simulink model "DvrSimKeybdCircuit_cs"  (R2016a)
settings: Solver=ode5  SolverMode=SingleTasking  StartTime=0.0  StopTime=inf  FixedStep=1/1000  RelTol=1e-3
PreLoadFcn:
  | mbxruntime.callbacks.PreLoadFcn(bdroot);
PostLoadFcn:
  | mbxruntime.callbacks.PostLoadFcn(bdroot);
InitFcn:
  | mbxruntime.callbacks.InitFcn(bdroot);
StartFcn:
  | mbxruntime.callbacks.StartFcn(bdroot);
StopFcn:
  | mbxruntime.callbacks.StopFcn(bdroot);
model workspace (MAT data in the model file):
  mbox_table : struct (value not decoded)
  model_closed = 0
  sim_status = 0
undefined symbols (not defined in the file or in its folder): BMotor1, BMotor2, BrkDelayTime, DControlB, Delay1, Delay2, DiscIntNeverNeededParam, IControlB, JMotor1, JMotor2, PControlB, PreScanCarSimLoadFcn, ratioGearF, ratioGearR, TorqDelayTime, Tstep
undefined symbols (not defined in the file): SteeringColumn, SteeringWheel, WheelL0, WheelL1, WheelR0, WheelR1
libraries: simulink x12, simulink_extras x5, MyLib x3, PreScanSimulinkLibrary x3, Solver_SF x2, pil_lib x1, PreScanUsefulBlocks x1
(part 4 of 9)

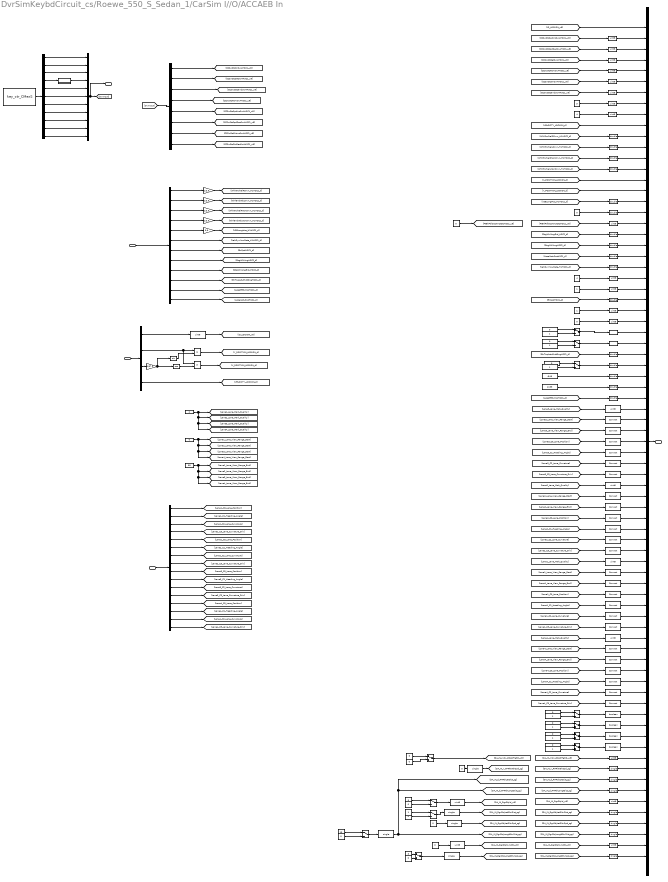
== system DvrSimKeybdCircuit_cs/Roewe_550_S_Sedan_1/CarSim I//O/ACCAEB In ==
  note: Here was constant 1, dont know why
  CarSimOut : Inport
  LanesInfo : Inport  Port=2
  LR_TIS : Inport  Port=3
  BrkPdlPos_H1HSC1_d1 : Constant  Value=0  OutDataTypeStr=double
  BrkPdlPos_H1HSC1_d2 : Constant  Value=0  OutDataTypeStr=uint8
  Bus Creator : BusCreator  Inputs=11
  Bus Creator1 : BusCreator  Inputs=77
  Bus Selector : BusSelector  OutputSignals=Lane1C0,Lane1C1,Lane1C2,Lane1C3,Lane2C0,Lane2C1,Lane2C2,Lane2C3,Lane3C0,Lane3C1,Lane3C2,Lane3C3,Lane4C0,Lane4C1,Lane4C2,Lane4C3
  Bus Selector1 : BusSelector  OutputSignals=WhlGndVelRDrvn_H1HSC2_d[km/h] (signal 38),WhlGndVelLDrvn_H1HSC2_d[km/h] (signal 39),WhlGndVelRNonDrvn_H1HSC2_d[km/h] (signal 40),WhlGndVelLNonDrvn_H1HSC2_d[km/h] (signal 41),VSELongtAcc_H1HSC1_d[g] (signal 42),VehDynYawRate_H1HSC1_d[deg/s] (signal 43),EnSpdHSC1_d[rpm] (signal 36),SteeringWheelAngle[deg] (signal 34),StrgWhlAngGrd_HSC2_d[deg/s] (signal 44),EnToqActuExtdRngHSC1_d[N M] (signal 37),AccelEfctvPosHSC1_d (signal 46),AccelActuPosHSC1_d (signal 45)
  Bus Selector2 : BusSelector  OutputSignals=ID ,Range ,Theta ,RlvSpd
  Bus Selector4 : BusSelector  OutputSignals=On,Set,Cancel,Resume,SpdInc,SpdDec,DisInc,DisDec
  Constant : Constant  Value=2
  Constant{1,93,102,104..105,107,110..111} (8 alike) : Constant  Value=0
  Constant{94,103,106,108..109,112..113} (7 alike) : Constant
  Constant2 : Constant  Value=95
  Constant3 : Constant  Value=1199
  Constant4 : Constant  Value=-848
  DA_IN_DgrObjSyncCtr_u1 : Constant  Value=0  OutDataTypeStr=uint8
  DA_IN_DgrObjSyncCtr_u2 : Constant  Value=0  OutDataTypeStr=uint8
  DA_IN_DgrObjSyncCtr_u3 : Constant  Value=0  OutDataTypeStr=uint8
  Data Type Conversion{,4..8,10..12,23,28..29,31..32,45,58,66,73,86,89,115,120,124} (23 alike) : DataTypeConversion  OutDataTypeStr=uint8
  Data Type Conversion{9,87..88,90..91,117..119,121..123,125} (12 alike) : DataTypeConversion  OutDataTypeStr=single
  Data Type Conversion{15..18,21..22,24..27,30,35..39} (16 alike) : DataTypeConversion  OutDataTypeStr=double
  Data Type Conversion{33..34,80..83} (6 alike) : DataTypeConversion  OutDataTypeStr=boolean
  Data Type Conversion{46..48,55..57,60..65,67..72,74..79} (24 alike) : DataTypeConversion
  Demux1 : Demux  Outputs=11
  DrvrSbltAtcHSC1_u1 : Constant  OutDataTypeStr=uint8
  EPBAppcnStsHSC1_u1 : Constant  Value=0  OutDataTypeStr=uint8
  EnTypHSC2_u1 : Constant  OutDataTypeStr=uint8
  FntLatDist10 : Constant  Value=0  OutDataTypeStr=double
      settings: AttributesFormatString=%<OutDataTypeStr>
  FntLatDist11 : Constant  Value=13  OutDataTypeStr=double
      settings: AttributesFormatString=%<OutDataTypeStr>
  FntLatDist12 : Constant  Value=0  OutDataTypeStr=double
      settings: AttributesFormatString=%<OutDataTypeStr>
  FntLatDist7 : Constant  Value=3  OutDataTypeStr=double
      settings: AttributesFormatString=%<OutDataTypeStr>
  FntLatDist8 : Constant  Value=0  OutDataTypeStr=double
      settings: AttributesFormatString=%<OutDataTypeStr>
  FntLatDist9 : Constant  OutDataTypeStr=double
      settings: AttributesFormatString=%<OutDataTypeStr>
  Gain{,1..3} (4 alike) : Gain  Gain=1/3.6
  Gain4 : Gain  Gain=9.8
  Gain5 : Gain  Gain=1/57.3
  ID_LOCKON_u5 : Constant  Value=5  OutDataTypeStr=uint8
  ID_LOCKON_u6 : Constant  Value=0  OutDataTypeStr=uint8
  ID_LOCKON_u7 : Constant  Value=5  OutDataTypeStr=uint8
  ID_LOCKON_u9 : Constant  Value=0  OutDataTypeStr=uint8
  Manual Switch{56,60..70} (12 alike) : ManualSwitch
  On Hold : Subsystem
  Product1 : Product
  Product2 : Product
  S-Function1 : S-Function  FunctionName=key_ctr_CMexS  SFunctionDeploymentMode=off  EnableBusSupport=off
  SysPwrMd_H1HSC1_u1 : Constant  Value=3  OutDataTypeStr=uint8
      settings: AttributesFormatString=%<DataType=%<OutDataTypeStr>>
  TrEstdGear_HSC1_u1 : Constant  Value=4  OutDataTypeStr=uint8
  TrShftLvrPosHSC1_u1 : Constant  Value=4  OutDataTypeStr=uint8
  Trigonometric Function : Trigonometry
  Trigonometric Function1 : Trigonometry  Operator=cos
  ACCAEBInput : Outport  OutDataTypeStr=Bus: AccAebInputs
  DvrInput : Outport  Port=2
  wires:
  LanesInfo/1 -> Bus Selector/1
  TrEstdGear_HSC1_u1/1 -> Data Type Conversion28/1  "TrEstdGear_HSC1_u8"
  [StrgWhlAngGrd_HSC2_d] -> Data Type Conversion24/1  "StrgWhlAngGrd_HSC2_d"
  [VELOCITY_LOCKON_d] -> Bus Creator1/10  "VELOCITY_LOCKON_d"
  [X_POSITION_LOCKON_d] -> Bus Creator1/15  "X_POSITION_LOCKON_d"
  [VehDynYawRate_H1HSC1_d] -> Data Type Conversion27/1
  [PtBrkPdlDscrtInptStsHSC1_u8] -> Data Type Conversion23/1  "PtBrkPdlDscrtInptStsHSC1_u8"
  BrkPdlPos_H1HSC1_d1/1 -> Data Type Conversion22/1  "BrkPdlPos_H1HSC1_d"
  TrShftLvrPosHSC1_u1/1 -> Data Type Conversion12/1  "TrShftLvrPosHSC1_u8"
  Bus Creator1/1 -> ACCAEBInput/1
  EnTypHSC2_u1/1 -> Data Type Conversion29/1  "EnTypHSC2_u8"
  DrvrSbltAtcHSC1_u1/1 -> Data Type Conversion31/1  "DrvrSbltAtcHSC1_u8"
  EPBAppcnStsHSC1_u1/1 -> Data Type Conversion32/1  "EPBAppcnStsHSC1_u8"
  SysPwrMd_H1HSC1_u1/1 -> Data Type Conversion11/1  "SysPwrMd_H1HSC1_u8"
  [VSELongtAcc_H1HSC1_d] -> Data Type Conversion21/1  "VSELongtAcc_H1HSC1_d"
  [StrgWhlAngHSC2_d] -> Data Type Conversion25/1  "StrgWhlAngHSC2_d"
  [WhlGndVelRDrvn_H1HSC2_d] -> Data Type Conversion15/1  "WhlGndVelRDrvn_H1HSC2_d"
  [WhlGndVelLDrvn_H1HSC2_d] -> Data Type Conversion16/1  "WhlGndVelLDrvn_H1HSC2_d"
  [WhlGndVelRNonDrvn_H1HSC2_d] -> Data Type Conversion17/1  "WhlGndVelRNonDrvn_H1HSC2_d"
  [WhlGndVelLNonDrvn_H1HSC2_d] -> Data Type Conversion18/1  "WhlGndVelLNonDrvn_H1HSC2_d"
  [EnSpdHSC1_d] -> Data Type Conversion30/1  "EnSpdHSC1_d"
  [Y_POSITION_LOCKON_d] -> Bus Creator1/16  "Y_POSITION_LOCKON_d"
  [CCSwStsSpdIncSwAHSC1_u8] -> Data Type Conversion4/1  "CCSwStsSpdIncSwAHSC1_u8"
  [CCSwStsSpdDecSwAHSC1_u8] -> Data Type Conversion5/1  "CCSwStsSpdDecSwAHSC1_u8"
  [CCSwStsSetSwAHSC1_u8] -> Data Type Conversion6/1  "CCSwStsSetSwAHSC1_u8"
  [CCSwStsRsmSwAHSC1_u8] -> Data Type Conversion7/1  "CCSwStsRsmSwAHSC1_u8"
  [CCSwStsOnSwAHSC1_u8] -> Data Type Conversion8/1  "CCSwStsOnSwAHSC1_u8"
  [CCSwStsCanclSwAHSC1_u8] -> Data Type Conversion10/1  "CCSwStsCanclSwAHSC1_u8"
  [AccelActuPosHSC1_d] -> Data Type Conversion26/1  "AccelActuPosHSC1_d"
  [EnToqActuExtdRngHSC1_d] -> Data Type Conversion35/1  "EnToqActuExtdRngHSC1_d"
  Manual Switch56/1 -> Data Type Conversion36/1
  Constant94/1 -> Manual Switch56/2
  Constant93/1 -> Manual Switch56/1
  Data Type Conversion36/1 -> Bus Creator1/32  "EnToqDrvrReqdExtdRngHSC1_d"
  Data Type Conversion37/1 -> Bus Creator1/33  "EnToqMinExtdRngHSC1_d"
  Data Type Conversion38/1 -> Bus Creator1/34  "EnToqMaxExtdRngHSC1_d"
  [AccelEfctvPosHSC1_d] -> Data Type Conversion39/1  "AccelEfctvPosHSC1_d"
  Data Type Conversion45/1 -> Bus Creator1/36  "Lane0_Lane_Mark_Quality"
  Data Type Conversion46/1 -> Bus Creator1/37  "Lane0_Lane_View_Range_Start"
  Data Type Conversion47/1 -> Bus Creator1/38  "Lane0_Lane_View_Range_End"
  Data Type Conversion48/1 -> Bus Creator1/39  "Lane0_C0_Lane_Position"
  Data Type Conversion55/1 -> Bus Creator1/40  "Lane0_C1_Heading_Angle"
  Data Type Conversion56/1 -> Bus Creator1/41  "Lane0_C2_Lane_Curvature"
  Data Type Conversion57/1 -> Bus Creator1/42  "Lane0_C3_Lane_Curvature_Driv"
  Data Type Conversion58/1 -> Bus Creator1/43  "Lane1_Lane_Mark_Quality"
  Data Type Conversion60/1 -> Bus Creator1/44  "Lane1_Lane_View_Range_Start"
  Data Type Conversion61/1 -> Bus Creator1/45  "Lane1_Lane_View_Range_End"
  Data Type Conversion62/1 -> Bus Creator1/46  "Lane1_C0_Lane_Position"
  Data Type Conversion63/1 -> Bus Creator1/47  "Lane1_C1_Heading_Angle"
  Data Type Conversion64/1 -> Bus Creator1/48  "Lane1_C2_Lane_Curvature"
  Data Type Conversion65/1 -> Bus Creator1/49  "Lane1_C3_Lane_Curvature_Driv"
  Data Type Conversion66/1 -> Bus Creator1/50  "Lane2_Lane_Mark_Quality"
  Data Type Conversion67/1 -> Bus Creator1/51  "Lane2_Lane_View_Range_Start"
  Data Type Conversion68/1 -> Bus Creator1/52  "Lane2_Lane_View_Range_End"
  Data Type Conversion69/1 -> Bus Creator1/53  "Lane2_C0_Lane_Position"
  Data Type Conversion70/1 -> Bus Creator1/54  "Lane2_C1_Heading_Angle"
  Data Type Conversion71/1 -> Bus Creator1/55  "Lane2_C2_Lane_Curvature"
  Data Type Conversion72/1 -> Bus Creator1/56  "Lane2_C3_Lane_Curvature_Driv"
  Manual Switch60/1 -> Data Type Conversion80/1
  Constant103/1 -> Manual Switch60/2
  Constant102/1 -> Manual Switch60/1
  Manual Switch63/1 -> Data Type Conversion81/1
  Constant109/1 -> Manual Switch63/2
  Constant104/1 -> Manual Switch63/1
  Manual Switch61/1 -> Data Type Conversion82/1
  Constant106/1 -> Manual Switch61/2
  Constant105/1 -> Manual Switch61/1
  Manual Switch62/1 -> Data Type Conversion83/1
  Constant108/1 -> Manual Switch62/2
  Constant107/1 -> Manual Switch62/1
  Data Type Conversion78/1 -> Bus Creator1/62  "Lane3_C2_Lane_Curvature"
  Data Type Conversion83/1 -> Bus Creator1/67  "MainBeamLghtOnHSC1"
  Data Type Conversion79/1 -> Bus Creator1/63  "Lane3_C3_Lane_Curvature_Driv"
  Data Type Conversion81/1 -> Bus Creator1/65  "FrtFogLghtOnHSC1"
  Data Type Conversion77/1 -> Bus Creator1/61  "Lane3_C1_Heading_Angle"
  Data Type Conversion82/1 -> Bus Creator1/66  "DipdBeamLghtOnHSC1"
  Data Type Conversion80/1 -> Bus Creator1/64  "RrFogLghtOnHSC1_b"
  Data Type Conversion75/1 -> Bus Creator1/59  "Lane3_Lane_View_Range_End"
  Data Type Conversion76/1 -> Bus Creator1/60  "Lane3_C0_Lane_Position"
  Data Type Conversion73/1 -> Bus Creator1/57  "Lane3_Lane_Mark_Quality"
  Data Type Conversion74/1 -> Bus Creator1/58  "Lane3_Lane_View_Range_Start"
  Manual Switch65/1 -> Data Type Conversion33/1
  Constant113/1 -> Manual Switch65/2
  Constant110/1 -> Manual Switch65/1
  Data Type Conversion33/1 -> Bus Creator1/29  "RDircnIOHSC1_b"
  Manual Switch64/1 -> Data Type Conversion34/1
  Constant112/1 -> Manual Switch64/2
  Constant111/1 -> Manual Switch64/1
  Data Type Conversion34/1 -> Bus Creator1/30  "LDircnIOHSC1_b"
  [DA_IN_indx_RCARrTgtID_u8] -> Data Type Conversion115/1  "DA_IN_indx_RCARrTgtID_u8"
  [DA_IN_v_RMRltVehSpd_sg] -> Data Type Conversion117/1  "DA_IN_v_RMRltVehSpd_sg"
  [DA_IN_d_RMRdrLongtDist_sg] -> Data Type Conversion119/1  "DA_IN_d_RMRdrLongtDist_sg"
  [DA_IN_DgrObjId_u8] -> Data Type Conversion120/1  "DA_IN_DgrObjId_u8"
  [DA_IN_DgrObjLatRltvDist_sg] -> Data Type Conversion121/1  "DA_IN_DgrObjLatRltvDist_sg"
  [DA_IN_DgrObjLatRltvSpd_sg] -> Data Type Conversion122/1  "DA_IN_DgrObjLatRltvSpd_sg"
  [DA_IN_DgrObjLongtRltvSpd_sg] -> Data Type Conversion125/1  "DA_IN_DgrObjLongtRltvSpd_sg"
  [DA_IN_DgrObjLongtRltvDist_sg] -> Data Type Conversion123/1  "DA_IN_DgrObjLongtRltvDist_sg"
  [DA_IN_DgrObjSyncCtr_u8] -> Data Type Conversion124/1  "DA_IN_DgrObjSyncCtr_u8"
  [DA_IN_d_RMRdrLatDist_sg] -> Data Type Conversion118/1  "DA_IN_d_RMRdrLatDist_sg"
  ID_LOCKON_u5/1 -> Manual Switch66/1
  ID_LOCKON_u6/1 -> Manual Switch66/2
  Manual Switch66/1 -> Data Type Conversion86/1
  ID_LOCKON_u7/1 -> Manual Switch67/1
  ID_LOCKON_u9/1 -> Manual Switch67/2
  Manual Switch67/1 -> [DA_IN_indx_RCARrTgtID_u8]
  Data Type Conversion86/1 -> [DA_IN_DgrObjId_u8]
  FntLatDist11/1 -> Manual Switch68/1
  FntLatDist12/1 -> Manual Switch68/2
  Manual Switch68/1 -> Data Type Conversion88/1
  FntLatDist9/1 -> Manual Switch69/1
  FntLatDist10/1 -> Manual Switch69/2
  Manual Switch69/1 -> Data Type Conversion87/1
  FntLatDist7/1 -> Manual Switch70/1
  FntLatDist8/1 -> Manual Switch70/2
  Manual Switch70/1 -> Data Type Conversion90/1
  DA_IN_DgrObjSyncCtr_u3/1 -> Data Type Conversion91/1
  Data Type Conversion87/1 -> [DA_IN_DgrObjLatRltvDist_sg]
  Data Type Conversion88/1 -> [DA_IN_DgrObjLongtRltvDist_sg], [DA_IN_d_RMRdrLongtDist_sg], [DA_IN_d_RMRdrLatDist_sg]
  Data Type Conversion89/1 -> [DA_IN_DgrObjSyncCtr_u8]
  Data Type Conversion90/1 -> [DA_IN_DgrObjLongtRltvSpd_sg]
  Data Type Conversion91/1 -> [DA_IN_v_RMRltVehSpd_sg]
  [ID_LOCKON_u8] -> Bus Creator1/1  "ID_LOCKON_u8"
  [Lane2_Lane_Mark_Quality] -> Data Type Conversion58/1
  [Lane2_Lane_View_Range_Start] -> Data Type Conversion60/1
  [Lane2_Lane_View_Range_End] -> Data Type Conversion61/1
  [Lane2_C0_Lane_Position] -> Data Type Conversion62/1
  [Lane2_C1_Heading_Angle] -> Data Type Conversion63/1
  [Lane2_C2_Lane_Curvature] -> Data Type Conversion64/1
  [Lane2_C3_Lane_Curvature_Driv] -> Data Type Conversion65/1
  [Lane4_Lane_Mark_Quality] -> Data Type Conversion73/1
  [Lane4_Lane_View_Range_Start] -> Data Type Conversion74/1
  [Lane4_Lane_View_Range_End] -> Data Type Conversion75/1
  [Lane4_C0_Lane_Position] -> Data Type Conversion76/1
  [Lane4_C1_Heading_Angle] -> Data Type Conversion77/1
  [Lane4_C2_Lane_Curvature] -> Data Type Conversion78/1
  [Lane4_C3_Lane_Curvature_Driv] -> Data Type Conversion79/1
  DA_IN_DgrObjSyncCtr_u1/1 -> Data Type Conversion9/1
  Data Type Conversion9/1 -> [DA_IN_DgrObjLatRltvSpd_sg]
  DA_IN_DgrObjSyncCtr_u2/1 -> Data Type Conversion89/1
  CarSimOut/1 -> Bus Selector1/1
  LR_TIS/1 -> Bus Selector2/1
  Bus Selector2/1 -> Data Type Conversion/1  "<ID >"
  Bus Selector2/4 -> [VELOCITY_LOCKON_d]  "<RlvSpd >"
  Constant/1 -> [Lane4_Lane_Mark_Quality], [Lane3_Lane_Mark_Quality], [Lane2_Lane_Mark_Quality], [Lane1_Lane_Mark_Quality]
  Constant1/1 -> [Lane4_Lane_View_Range_Start], [Lane3_Lane_View_Range_Start], [Lane2_Lane_View_Range_Start], [Lane1_Lane_View_Range_Start]
  Constant2/1 -> [Lane4_Lane_View_Range_End], [Lane3_Lane_View_Range_End], [Lane2_Lane_View_Range_End], [Lane1_Lane_View_Range_End]
  Bus Selector1/1 -> Gain/1  "<WhlGndVelRDrvn_H1HSC2_d[km/h] (signal 38)>"
  Bus Selector1/2 -> Gain1/1  "<WhlGndVelLDrvn_H1HSC2_d[km/h] (signal 39)>"
  Bus Selector1/3 -> Gain2/1  "<WhlGndVelRNonDrvn_H1HSC2_d[km/h] (signal 40)>"
  Bus Selector1/4 -> Gain3/1  "<WhlGndVelLNonDrvn_H1HSC2_d[km/h] (signal 41)>"
  Bus Selector1/5 -> Gain4/1  "<VSELongtAcc_H1HSC1_d[g] (signal 42)>"
  Bus Selector1/6 -> [VehDynYawRate_H1HSC1_d]  "<VehDynYawRate_H1HSC1_d[deg/s] (signal 43)>"
  Bus Selector1/7 -> [EnSpdHSC1_d]  "<EnSpdHSC1_d[rpm] (signal 36)>"
  Bus Selector1/8 -> [StrgWhlAngHSC2_d]  "<SteeringWheelAngle[deg] (signal 34)>"
  Bus Selector1/9 -> [StrgWhlAngGrd_HSC2_d]  "<StrgWhlAngGrd_HSC2_d[deg/s] (signal 44)>"
  Gain/1 -> [WhlGndVelRDrvn_H1HSC2_d]
  Gain1/1 -> [WhlGndVelLDrvn_H1HSC2_d]
  Gain2/1 -> [WhlGndVelRNonDrvn_H1HSC2_d]
  Gain3/1 -> [WhlGndVelLNonDrvn_H1HSC2_d]
  Gain4/1 -> [VSELongtAcc_H1HSC1_d]
  Constant3/1 -> Data Type Conversion38/1
  Constant4/1 -> Data Type Conversion37/1
  Bus Selector1/12 -> [AccelActuPosHSC1_d]  "<AccelActuPosHSC1_d (signal 45)>"
  Bus Selector1/11 -> [AccelEfctvPosHSC1_d]  "<AccelEfctvPosHSC1_d (signal 46)>"
  Bus Selector1/10 -> [EnToqActuExtdRngHSC1_d]  "<EnToqActuExtdRngHSC1_d[N M] (signal 37)>"
  BrkPdlPos_H1HSC1_d2/1 -> [PtBrkPdlDscrtInptStsHSC1_u8]
  Bus Selector4/5 -> [CCSwStsSpdIncSwAHSC1_u8]  "<SpdInc>"
  Data Type Conversion/1 -> [ID_LOCKON_u8]
  Data Type Conversion4/1 -> Bus Creator1/2  "CCSwStsSpdIncSwAHSC1_u8"
  Data Type Conversion5/1 -> Bus Creator1/3  "CCSwStsSpdDecSwAHSC1_u8"
  Data Type Conversion6/1 -> Bus Creator1/4  "CCSwStsSetSwAHSC1_u8"
  Data Type Conversion7/1 -> Bus Creator1/5  "CCSwStsRsmSwAHSC1_u8"
  Data Type Conversion8/1 -> Bus Creator1/6  "CCSwStsOnSwAHSC1_u8"
  Data Type Conversion10/1 -> Bus Creator1/7  "CCSwStsCanclSwAHSC1_u8"
  Data Type Conversion11/1 -> Bus Creator1/8  "SysPwrMd_H1HSC1_u8"
  Data Type Conversion12/1 -> Bus Creator1/9  "TrShftLvrPosHSC1_u8"
  Data Type Conversion15/1 -> Bus Creator1/11  "WhlGndVelRDrvn_H1HSC2_d"
  Data Type Conversion16/1 -> Bus Creator1/12  "WhlGndVelLDrvn_H1HSC2_d"
  Data Type Conversion17/1 -> Bus Creator1/13  "WhlGndVelRNonDrvn_H1HSC2_d"
  Data Type Conversion18/1 -> Bus Creator1/14  "WhlGndVelLNonDrvn_H1HSC2_d"
  Data Type Conversion21/1 -> Bus Creator1/17  "VSELongtAcc_H1HSC1_d"
  Data Type Conversion22/1 -> Bus Creator1/18  "BrkPdlPos_H1HSC1_d"
  Data Type Conversion23/1 -> Bus Creator1/19  "PtBrkPdlDscrtInptStsHSC1_u8"
  Data Type Conversion24/1 -> Bus Creator1/20  "StrgWhlAngGrd_HSC2_d"
  Data Type Conversion25/1 -> Bus Creator1/21  "StrgWhlAngHSC2_d"
  Data Type Conversion26/1 -> Bus Creator1/22  "AccelActuPosHSC1_d"
  Data Type Conversion27/1 -> Bus Creator1/23  "VehDynYawRate_H1HSC1_d"
  Data Type Conversion28/1 -> Bus Creator1/24  "TrEstdGear_HSC1_u8"
  Data Type Conversion29/1 -> Bus Creator1/25  "EnTypHSC2_u8"
  Data Type Conversion30/1 -> Bus Creator1/26  "EnSpdHSC1_d"
  Data Type Conversion31/1 -> Bus Creator1/27  "DrvrSbltAtcHSC1_u8"
  Data Type Conversion32/1 -> Bus Creator1/28  "EPBAppcnStsHSC1_u8"
  Data Type Conversion35/1 -> Bus Creator1/31  "EnToqActuExtdRngHSC1_d"
  Data Type Conversion39/1 -> Bus Creator1/35  "AccelEfctvPosHSC1_d"
  Data Type Conversion115/1 -> Bus Creator1/68  "DA_IN_indx_RCARrTgtID_u8"
  Data Type Conversion117/1 -> Bus Creator1/69  "DA_IN_v_RMRltVehSpd_sg"
  Data Type Conversion118/1 -> Bus Creator1/70  "DA_IN_d_RMRdrLatDist_sg"
  Data Type Conversion119/1 -> Bus Creator1/71  "DA_IN_d_RMRdrLongtDist_sg"
  Data Type Conversion120/1 -> Bus Creator1/72  "DA_IN_DgrObjId_u8"
  Data Type Conversion121/1 -> Bus Creator1/73  "DA_IN_DgrObjLatRltvDist_sg"
  Data Type Conversion122/1 -> Bus Creator1/74  "DA_IN_DgrObjLatRltvSpd_sg"
  Data Type Conversion123/1 -> Bus Creator1/75  "DA_IN_DgrObjLongtRltvDist_sg"
  Data Type Conversion124/1 -> Bus Creator1/76  "DA_IN_DgrObjSyncCtr_u8"
  Data Type Conversion125/1 -> Bus Creator1/77  "DA_IN_DgrObjLongtRltvSpd_sg"
  Bus Selector/12 -> [Lane3_C3_Lane_Curvature_Driv]  "<Lane3C3>"
  Bus Selector/14 -> [Lane4_C1_Heading_Angle]  "<Lane4C1>"
  Bus Selector/10 -> [Lane3_C1_Heading_Angle]  "<Lane3C1>"
  Bus Selector/4 -> [Lane1_C3_Lane_Curvature_Driv]  "<Lane1C3>"
  Bus Selector/8 -> [Lane2_C3_Lane_Curvature_Driv]  "<Lane2C3>"
  Bus Selector/7 -> [Lane2_C2_Lane_Curvature]  "<Lane2C2>"
  Bus Selector/1 -> [Lane1_C0_Lane_Position]  "<Lane1C0>"
  Bus Selector/15 -> [Lane4_C2_Lane_Curvature]  "<Lane4C2>"
  Bus Selector/3 -> [Lane1_C2_Lane_Curvature]  "<Lane1C2>"
  Bus Selector/11 -> [Lane3_C2_Lane_Curvature]  "<Lane3C2>"
  Bus Selector/16 -> [Lane4_C3_Lane_Curvature_Driv]  "<Lane4C3>"
  Bus Selector/2 -> [Lane1_C1_Heading_Angle]  "<Lane1C1>"
  Bus Selector/5 -> [Lane2_C0_Lane_Position]  "<Lane2C0>"
  Bus Selector/13 -> [Lane4_C0_Lane_Position]  "<Lane4C0>"
  Bus Selector/9 -> [Lane3_C0_Lane_Position]  "<Lane3C0>"
  Bus Selector/6 -> [Lane2_C1_Heading_Angle]  "<Lane2C1>"
  [Lane3_Lane_Mark_Quality] -> Data Type Conversion45/1
  [Lane3_Lane_View_Range_Start] -> Data Type Conversion46/1
  [Lane3_Lane_View_Range_End] -> Data Type Conversion47/1
  [Lane3_C0_Lane_Position] -> Data Type Conversion48/1
  [Lane3_C1_Heading_Angle] -> Data Type Conversion55/1
  [Lane3_C2_Lane_Curvature] -> Data Type Conversion56/1
  [Lane3_C3_Lane_Curvature_Driv] -> Data Type Conversion57/1
  [Lane1_Lane_Mark_Quality] -> Data Type Conversion66/1
  [Lane1_Lane_View_Range_Start] -> Data Type Conversion67/1
  [Lane1_Lane_View_Range_End] -> Data Type Conversion68/1
  [Lane1_C0_Lane_Position] -> Data Type Conversion69/1
  [Lane1_C1_Heading_Angle] -> Data Type Conversion70/1
  [Lane1_C2_Lane_Curvature] -> Data Type Conversion71/1
  [Lane1_C3_Lane_Curvature_Driv] -> Data Type Conversion72/1
  Bus Selector4/2 -> [CCSwStsSetSwAHSC1_u8]  "<Set>"
  S-Function1/1 -> Demux1/1
  Demux1/5 -> Bus Creator/5  "Set"
  Demux1/6 -> Bus Creator/6  "Cancel"
  Demux1/7 -> Bus Creator/7  "Resume"
  Demux1/8 -> Bus Creator/8  "SpdInc"
  Demux1/9 -> Bus Creator/9  "SpdDec"
  Demux1/10 -> Bus Creator/10  "DisInc"
  Demux1/11 -> Bus Creator/11  "DisDec"
  Demux1/3 -> Bus Creator/3  "DrvBrake"
  Demux1/2 -> Bus Creator/2  "DrvAngle"
  Demux1/1 -> Bus Creator/1  "DvrThrottle"
  Demux1/4 -> On Hold/1(In1)
  On Hold/1(Out1) -> Bus Creator/4  "On"
  [DvrInput] -> Bus Selector4/1
  Bus Selector4/1 -> [CCSwStsOnSwAHSC1_u8]  "<On>"
  Bus Selector4/3 -> [CCSwStsCanclSwAHSC1_u8]  "<Cancel>"
  Bus Selector4/4 -> [CCSwStsRsmSwAHSC1_u8]  "<Resume>"
  Bus Selector4/6 -> [CCSwStsSpdDecSwAHSC1_u8]  "<SpdDec>"
  Bus Creator/1 -> [DvrInput], DvrInput/1
  Bus Selector2/3 -> Gain5/1  "<Theta >"
  Trigonometric Function/1 -> Product1/2
  Bus Selector2/2 -> Product2/1, Product1/1  "<Range >"
  Trigonometric Function1/1 -> Product2/2
  Product2/1 -> [X_POSITION_LOCKON_d]
  Product1/1 -> [Y_POSITION_LOCKON_d]
  Gain5/1 -> Trigonometric Function/1, Trigonometric Function1/1
  Bus Selector4/7 -> [CCSwStsDisIncSwAHSC1_u8]  "<DisInc>"
  Bus Selector4/8 -> [CCSwStsDisDecSwAHSC1_u8]  "<DisDec>"

== system DvrSimKeybdCircuit_cs/Roewe_550_S_Sedan_1/CarSim I//O/Actors ==
  DCUOut : Inport
  CarSimOut : Inport  Port=2
  DvrInput : Inport  Port=3
  AX_Tartget : Scope
  Bus Creator1 : BusCreator  Inputs=5
  Bus Selector : BusSelector  OutputSignals=ACCSysSts_RadarHSC2_u8,ACCToqReqValHSC2_sg,ACCAccReqValHSC2_sg
  Bus Selector2 : BusSelector  OutputSignals=AV_D3f (signal 57),AV_D3r (signal 58),Ax_SM[g] (signal 54)
  Bus Selector4 : BusSelector  OutputSignals=DvrThrottle,DrvBrake
  Bus Selector5 : BusSelector  OutputSignals=DrvAngle,DvrThrottle
  Constant1 : Constant  Value=2
  Demux : Demux  Outputs=2
  Gain : Gain  Gain=4
  Gain1 : Gain
  Gain2 : Gain  Gain=350
  Gain3 : Gain  Gain=-0.08
  LongExecutor : Subsystem
  MF : Scope
  Mux : Mux  Inputs=2
  Mux1 : Mux  Inputs=2
  P_BK : Scope
  Subtract : Sum  Inputs=+-
  Switch : Switch  Criteria=u2 ~= 0
  T_Target : Scope
  CarSimProcCtrl : Outport
  wires:
  Bus Selector4/1 -> Gain2/1  "<DvrThrottle>"
  LongExecutor/1(PCON_BK) -> P_BK/1, Bus Creator1/3  "Pcon_BK"
  LongExecutor/3(M_OUT_D3_R) -> Bus Creator1/5  "M_OUT_D3_R"
  LongExecutor/2(M_OUT_D3_F) -> MF/1, Bus Creator1/4  "M_OUT_D3_F"
  Bus Selector5/1 -> Bus Creator1/1  "<DrvAngle>"
  Bus Creator1/1 -> CarSimProcCtrl/1
  Bus Selector2/1 -> LongExecutor/3(AV_D3f)  "<AV_D3f (signal 57)>"
  Bus Selector2/2 -> LongExecutor/4(AV_D3r)  "<AV_D3r (signal 58)>"
  Bus Selector2/3 -> LongExecutor/5(Ax)  "<Ax_SM[g] (signal 54)>"
  Switch/1 -> Demux/1
  Demux/1 -> T_Target/1, LongExecutor/1(T_Target)
  Demux/2 -> AX_Tartget/1, LongExecutor/2(AxTarget)
  DCUOut/1 -> [DCUOut]
  CarSimOut/1 -> [CarSimOut]
  [CarSimOut] -> Bus Selector2/1
  Bus Selector/1 -> Subtract/1  "<ACCSysSts_RadarHSC2_u8>"
  Subtract/1 -> Switch/2
  Constant1/1 -> Subtract/2
  Bus Selector/2 -> Gain/1  "<ACCToqReqValHSC2_sg>"
  Bus Selector/3 -> Gain1/1  "<ACCAccReqValHSC2_sg>"
  Mux/1 -> Switch/3
  [DCUOut] -> Bus Selector/1
  Gain/1 -> Mux/1
  Gain1/1 -> Mux/2
  DvrInput/1 -> [DvrInput]
  [DvrInput] -> Bus Selector4/1
  Bus Selector4/2 -> Gain3/1  "<DrvBrake>"
  Mux1/1 -> Switch/1
  Gain2/1 -> Mux1/1
  Gain3/1 -> Mux1/2
  [DvrInput] -> Bus Selector5/1
  Bus Selector5/2 -> Bus Creator1/2  "<DvrThrottle>"

== system DvrSimKeybdCircuit_cs/Roewe_550_S_Sedan_1/CarSim I//O/CarSim Status  ==
  PreScanInputs : Inport
  CarSimProcCtrl : Inport  Port=2
  Bus Creator1 : BusCreator  Inputs=67
  Bus Selector : BusSelector  OutputSignals=DrvAngle,DvrThrottle,Pcon_BK
  Bus Selector1 : BusSelector  OutputSignals=M_OUT_D3_F,M_OUT_D3_R
  CarSim S-Function2 : Solver_SF/CarSim S-Function2  Priority=1  VehicleCode=i_i  SIMFILE=simfile.sim
      settings: AttributesFormatString=Vehicle Code: %<VehicleCode>
  Constant : Constant  Value=0
  Demux : Demux  Outputs=67
  Display : Display
  Memory : Memory
  Mux : Mux  Inputs=8
  Mux1 : Mux  Inputs=3
  Scope : Scope
  Scope1 : Scope
  Subtract : Sum  Inputs=+-
  CarSimOut : Outport
  wires:
  CarSim S-Function2/1 -> Demux/1
  Mux/1 -> Memory/1
  Memory/1 -> CarSim S-Function2/1
  Bus Creator1/1 -> CarSimOut/1
  PreScanInputs/1 -> Mux/2
  CarSimProcCtrl/1 -> Bus Selector1/1, Bus Selector/1
  Bus Selector/1 -> Mux1/1  "<DrvAngle>"
  Bus Selector/2 -> Mux1/2  "<DvrThrottle>"
  Bus Selector/3 -> Mux1/3  "<Pcon_BK>"
  Mux1/1 -> Mux/1
  Bus Selector1/1 -> Mux/3  "<M_OUT_D3_F>"
  Bus Selector1/2 -> Mux/4  "<M_OUT_D3_R>"
  Demux/11 -> Bus Creator1/11  "CarSim_Pos_Wheel_FL_y[m]"
  Demux/14 -> Bus Creator1/14  "CarSim_Pos_Wheel_FR_y[m]"
  Demux/15 -> Bus Creator1/15  "CarSim_Pos_Wheel_FR_z[m]"
  Demux/16 -> Subtract/2, Bus Creator1/16  "CarSim_Pos_Wheel_RL_x[m]"
  Demux/19 -> Bus Creator1/19  "CarSim_Pos_Wheel_RR_x[m]"
  Demux/21 -> Scope/1, Bus Creator1/21  "CarSim_Pos_Wheel_RR_z[m]"
  Demux/12 -> Bus Creator1/12  "CarSim_Pos_Wheel_FL_z[m]"
  Demux/17 -> Bus Creator1/17  "CarSim_Pos_Wheel_RL_y[m]"
  Demux/9 -> Bus Creator1/9  "SprungMass_Angle_Global_Yaw[deg]"
  Demux/23 -> Bus Creator1/23  "CarSim_Angle_Wheel_FL_Rot[rev]"
  Demux/25 -> Bus Creator1/25  "CarSim_Angle_Wheel_FR_Roll[deg]"
  Demux/26 -> Bus Creator1/26  "CarSim_Angle_Wheel_FR_Rot[rev]"
  Demux/4 -> Bus Creator1/4  "VehicleCoG_Vx[km/h]"
  Demux/8 -> Bus Creator1/8  "SprungMass_Angle_Global_Pitch[deg]"
  Demux/10 -> Subtract/1, Bus Creator1/10  "CarSim_Pos_Wheel_FL_x[m]"
  Demux/2 -> Bus Creator1/2  "SprungMass_Pos_Global_y[m]"
  Demux/22 -> Bus Creator1/22  "CarSim_Angle_Wheel_FL_Roll[deg]"
  Demux/24 -> Bus Creator1/24  "CarSim_Angle_Wheel_FL_Steer[deg]"
  Demux/27 -> Bus Creator1/27  "CarSim_Angle_Wheel_FR_Steer[deg]"
  Demux/28 -> Bus Creator1/28  "CarSim_Angle_Wheel_RL_Roll[deg]"
  Demux/6 -> Bus Creator1/6  "VehicleCoG_Vz[km/h]"
  Demux/7 -> Bus Creator1/7  "SprungMass_Angle_Global_Roll[deg]"
  Demux/13 -> Bus Creator1/13  "CarSim_Pos_Wheel_FR_x[m]"
  Demux/18 -> Bus Creator1/18  "CarSim_Pos_Wheel_RL_Z[m]"
  Demux/20 -> Bus Creator1/20  "CarSim_Pos_Wheel_RR_y[m]"
  Demux/30 -> Bus Creator1/30  "CarSim_Angle_Wheel_RL_Steer[deg]"
  Demux/3 -> Scope1/1, Bus Creator1/3  "SprungMass_Pos_Global_z[m]"
  Demux/29 -> Bus Creator1/29  "CarSim_Angle_Wheel_RL_Rot[rev]"
  Demux/1 -> Bus Creator1/1  "SprungMass_Pos_Global_x[m]"
  Demux/5 -> Bus Creator1/5  "VehicleCoG_Vy[km/h]"
  Demux/48 -> Bus Creator1/48  "Mz_Kp_L1[NM]"
  Demux/52 -> Bus Creator1/52  "F_TRdL1[N]"
  Demux/59 -> Bus Creator1/59  "Reserved1"
  Demux/42 -> Bus Creator1/42  "VSELongtAcc_H1HSC1_d[g]"
  Demux/36 -> Bus Creator1/36  "EnSpdHSC1_d[rpm]"
  Demux/35 -> Bus Creator1/35  "Axle1ReducedSW"
  Demux/41 -> Bus Creator1/41  "WhlGndVelLNonDrvn_H1HSC2_d[km/h]"
  Demux/40 -> Bus Creator1/40  "WhlGndVelRNonDrvn_H1HSC2_d[km/h]"
  Demux/33 -> Bus Creator1/33  "CarSim_Angle_Wheel_RR_Steer[deg]"
  Demux/39 -> Bus Creator1/39  "WhlGndVelLDrvn_H1HSC2_d[km/h]"
  Demux/54 -> Bus Creator1/54  "Ax_SM[g]"
  Demux/61 -> Bus Creator1/61  "Reserved3"
  Demux/62 -> Bus Creator1/62  "Reserved4"
  Demux/46 -> Bus Creator1/46  "AccelEfctvPosHSC1_d"
  Demux/56 -> Bus Creator1/56  "GearStatus"
  Demux/63 -> Bus Creator1/63  "Reserved5"
  Demux/43 -> Bus Creator1/43  "VehDynYawRate_H1HSC1_d[deg/s]"
  Demux/58 -> Bus Creator1/58  "AV_D3r"
  Demux/65 -> Bus Creator1/65  "Reserved7"
  Demux/67 -> Bus Creator1/67  "Reserved9"
  Demux/32 -> Bus Creator1/32  "CarSim_Angle_Wheel_RR_Rot[rev]"
  Demux/47 -> Bus Creator1/47  "Pbk_Con[MPa]"
  Demux/66 -> Bus Creator1/66  "Reserved8"
  Demux/50 -> Bus Creator1/50  "Steer_L1[deg]"
  Demux/51 -> Bus Creator1/51  "Steer_R1[deg]"
  Demux/57 -> Bus Creator1/57  "AV_D3f"
  Demux/49 -> Bus Creator1/49  "Mz_Kp_L1[NM]"
  Demux/37 -> Bus Creator1/37  "EnToqActuExtdRngHSC1_d[N M]"
  Demux/38 -> Bus Creator1/38  "WhlGndVelRDrvn_H1HSC2_d[km/h]"
  Demux/34 -> Bus Creator1/34  "SteeringWheelAngle[deg]"
  Demux/53 -> Bus Creator1/53  "F_TRdR1[N]"
  Demux/44 -> Bus Creator1/44  "StrgWhlAngGrd_HSC2_d[deg/s]"
  Demux/45 -> Bus Creator1/45  "AccelActuPosHSC1_d"
  Demux/55 -> Bus Creator1/55  "Ay_SM[g]"
  Demux/60 -> Bus Creator1/60  "Reserved2"
  Demux/64 -> Bus Creator1/64  "Reserved6"
  Demux/31 -> Bus Creator1/31  "CarSim_Angle_Wheel_RR_Roll[deg]"
  Constant/1 -> Mux/8, Mux/7, Mux/6, Mux/5
  Subtract/1 -> Display/1

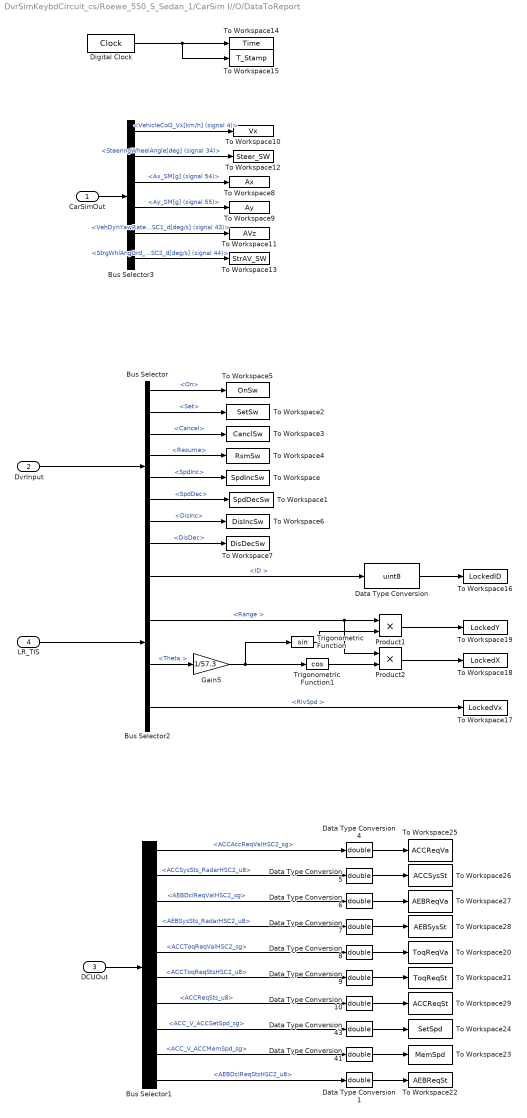
== system DvrSimKeybdCircuit_cs/Roewe_550_S_Sedan_1/CarSim I//O/DataToReport ==
  CarSimOut : Inport
  DvrInput : Inport  Port=2
  DCUOut : Inport  Port=3
  LR_TIS : Inport  Port=4
  Bus Selector : BusSelector  OutputSignals=On,Set,Cancel,Resume,SpdInc,SpdDec,DisInc,DisDec
  Bus Selector1 : BusSelector  OutputSignals=ACCAccReqValHSC2_sg,ACCSysSts_RadarHSC2_u8,AEBDclReqValHSC2_sg,AEBSysSts_RadarHSC2_u8,ACCToqReqValHSC2_sg,ACCToqReqStsHSC2_u8,ACCReqSts_u8,ACC_V_ACCSetSpd_sg,ACC_V_ACCMemSpd_sg,AEBDclReqStsHSC2_u8
  Bus Selector2 : BusSelector  OutputSignals=ID ,Range ,Theta ,RlvSpd
  Bus Selector3 : BusSelector  OutputSignals=VehicleCoG_Vx[km/h] (signal 4),SteeringWheelAngle[deg] (signal 34),Ax_SM[g] (signal 54),Ay_SM[g] (signal 55),VehDynYawRate_H1HSC1_d[deg/s] (signal 43),StrgWhlAngGrd_HSC2_d[deg/s] (signal 44)
  Data Type Conversion : DataTypeConversion  OutDataTypeStr=uint8
  Data Type Conversion{1,4..10,41,43} (10 alike) : DataTypeConversion  OutDataTypeStr=double
  Digital Clock : DigitalClock  SampleTime=0.05
  Gain5 : Gain  Gain=1/57.3
  Product1 : Product
  Product2 : Product
  To Workspace : ToWorkspace  VariableName=SpdIncSw  SampleTime=-1
  To Workspace1 : ToWorkspace  VariableName=SpdDecSw  SampleTime=-1
  To Workspace10 : ToWorkspace  VariableName=Vx  SampleTime=-1
  To Workspace11 : ToWorkspace  VariableName=AVz  SampleTime=-1
  To Workspace12 : ToWorkspace  VariableName=Steer_SW  SampleTime=-1
  To Workspace13 : ToWorkspace  VariableName=StrAV_SW  SampleTime=-1
  To Workspace14 : ToWorkspace  VariableName=Time  SampleTime=-1
  To Workspace15 : ToWorkspace  VariableName=T_Stamp  SampleTime=-1
  To Workspace16 : ToWorkspace  VariableName=LockedID  SampleTime=-1
  To Workspace17 : ToWorkspace  VariableName=LockedVx  SampleTime=-1
  To Workspace18 : ToWorkspace  VariableName=LockedX  SampleTime=-1
  To Workspace19 : ToWorkspace  VariableName=LockedY  SampleTime=-1
  To Workspace2 : ToWorkspace  VariableName=SetSw  SampleTime=-1
  To Workspace20 : ToWorkspace  VariableName=ToqReqVa  SampleTime=-1
  To Workspace21 : ToWorkspace  VariableName=ToqReqSt  SampleTime=-1
  To Workspace22 : ToWorkspace  VariableName=AEBReqSt  SampleTime=-1
  To Workspace23 : ToWorkspace  VariableName=MemSpd  SampleTime=-1
  To Workspace24 : ToWorkspace  VariableName=SetSpd  SampleTime=-1
  To Workspace25 : ToWorkspace  VariableName=ACCReqVa  SampleTime=-1
  To Workspace26 : ToWorkspace  VariableName=ACCSysSt  SampleTime=-1
  To Workspace27 : ToWorkspace  VariableName=AEBReqVa  SampleTime=-1
  To Workspace28 : ToWorkspace  VariableName=AEBSysSt  SampleTime=-1
  To Workspace29 : ToWorkspace  VariableName=ACCReqSt  SampleTime=-1
  To Workspace3 : ToWorkspace  VariableName=CanclSw  SampleTime=-1
  To Workspace4 : ToWorkspace  VariableName=RsmSw  SampleTime=-1
  To Workspace5 : ToWorkspace  VariableName=OnSw  SampleTime=-1
  To Workspace6 : ToWorkspace  VariableName=DisIncSw  SampleTime=-1
  To Workspace7 : ToWorkspace  VariableName=DisDecSw  SampleTime=-1
  To Workspace8 : ToWorkspace  VariableName=Ax  SampleTime=-1
  To Workspace9 : ToWorkspace  VariableName=Ay  SampleTime=-1
  Trigonometric Function : Trigonometry
  Trigonometric Function1 : Trigonometry  Operator=cos
  wires:
  Bus Selector/1 -> To Workspace5/1  "<On>"
  Bus Selector/3 -> To Workspace3/1  "<Cancel>"
  Bus Selector1/1 -> Data Type Conversion4/1  "<ACCAccReqValHSC2_sg>"
  Bus Selector1/2 -> Data Type Conversion5/1  "<ACCSysSts_RadarHSC2_u8>"
  Bus Selector1/3 -> Data Type Conversion6/1  "<AEBDclReqValHSC2_sg>"
  Bus Selector1/4 -> Data Type Conversion7/1  "<AEBSysSts_RadarHSC2_u8>"
  Bus Selector1/5 -> Data Type Conversion8/1  "<ACCToqReqValHSC2_sg>"
  Bus Selector1/6 -> Data Type Conversion9/1  "<ACCToqReqStsHSC2_u8>"
  Bus Selector1/7 -> Data Type Conversion10/1  "<ACCReqSts_u8>"
  Data Type Conversion4/1 -> To Workspace25/1
  Data Type Conversion5/1 -> To Workspace26/1
  Data Type Conversion6/1 -> To Workspace27/1
  Data Type Conversion7/1 -> To Workspace28/1
  Data Type Conversion8/1 -> To Workspace20/1
  Data Type Conversion9/1 -> To Workspace21/1
  Data Type Conversion10/1 -> To Workspace29/1
  Bus Selector1/8 -> Data Type Conversion43/1  "<ACC_V_ACCSetSpd_sg>"
  Data Type Conversion41/1 -> To Workspace23/1
  Data Type Conversion43/1 -> To Workspace24/1
  Bus Selector1/9 -> Data Type Conversion41/1  "<ACC_V_ACCMemSpd_sg>"
  Bus Selector1/10 -> Data Type Conversion1/1  "<AEBDclReqStsHSC2_u8>"
  Data Type Conversion1/1 -> To Workspace22/1
  DCUOut/1 -> Bus Selector1/1
  DvrInput/1 -> Bus Selector/1
  Bus Selector/2 -> To Workspace2/1  "<Set>"
  Bus Selector/4 -> To Workspace4/1  "<Resume>"
  Bus Selector/5 -> To Workspace/1  "<SpdInc>"
  Bus Selector/6 -> To Workspace1/1  "<SpdDec>"
  Bus Selector/8 -> To Workspace7/1  "<DisDec>"
  Bus Selector/7 -> To Workspace6/1  "<DisInc>"
  LR_TIS/1 -> Bus Selector2/1
  Bus Selector2/4 -> To Workspace17/1  "<RlvSpd >"
  Trigonometric Function/1 -> Product1/2
  Trigonometric Function1/1 -> Product2/2
  Gain5/1 -> Trigonometric Function/1, Trigonometric Function1/1
  Bus Selector2/1 -> Data Type Conversion/1  "<ID >"
  Bus Selector2/2 -> Product2/1, Product1/1  "<Range >"
  Bus Selector2/3 -> Gain5/1  "<Theta >"
  Data Type Conversion/1 -> To Workspace16/1
  Product1/1 -> To Workspace19/1
  Product2/1 -> To Workspace18/1
  CarSimOut/1 -> Bus Selector3/1
  Bus Selector3/1 -> To Workspace10/1  "<VehicleCoG_Vx[km/h] (signal 4)>"
  Bus Selector3/3 -> To Workspace8/1  "<Ax_SM[g] (signal 54)>"
  Bus Selector3/2 -> To Workspace12/1  "<SteeringWheelAngle[deg] (signal 34)>"
  Bus Selector3/4 -> To Workspace9/1  "<Ay_SM[g] (signal 55)>"
  Bus Selector3/5 -> To Workspace11/1  "<VehDynYawRate_H1HSC1_d[deg/s] (signal 43)>"
  Bus Selector3/6 -> To Workspace13/1  "<StrgWhlAngGrd_HSC2_d[deg/s] (signal 44)>"
  Digital Clock/1 -> To Workspace15/1, To Workspace14/1

== system DvrSimKeybdCircuit_cs/Roewe_550_S_Sedan_1/CarSim I//O/LaneMarker ==
  note: LiYong
  PreScanLaneMarker1 : Inport
  PreScanLaneMarker2 : Inport  Port=2
  PreScanLaneMarker3 : Inport  Port=3
  PreScanLaneMarker4 : Inport  Port=4
  PreScanLaneMarker5 : Inport  Port=5
  Bus Creator : BusCreator  Inputs=16
  Demux{1..4} (4 alike) : Demux
  MATLAB Function : MATLAB Function  TreatAsAtomicUnit=on
  Subsystem : Subsystem
  LanesInfo : Outport
  wires:
  PreScanLaneMarker1/1 -> Subsystem/1(LaneMarkerInfo)
  Demux1/2 -> Bus Creator/2  "Lane1C1"
  Demux2/4 -> Bus Creator/8  "Lane2C3"
  Demux2/3 -> Bus Creator/7  "Lane2C2"
  Demux3/4 -> Bus Creator/12  "Lane3C3"
  Demux2/2 -> Bus Creator/6  "Lane2C1"
  Demux3/3 -> Bus Creator/11  "Lane3C2"
  Demux4/4 -> Bus Creator/16  "Lane4C3"
  PreScanLaneMarker3/1 -> Subsystem/3(LaneMarkerInfo2)
  PreScanLaneMarker4/1 -> Subsystem/4(LaneMarkerInfo3)
  PreScanLaneMarker5/1 -> Subsystem/5(LaneMarkerInfo4)
  Subsystem/5(Lane2_X) -> MATLAB Function/5(Lane2_X)
  Bus Creator/1 -> LanesInfo/1
  Demux4/3 -> Bus Creator/15  "Lane4C2"
  Demux1/3 -> Bus Creator/3  "Lane1C2"
  Demux4/1 -> Bus Creator/13  "Lane4C0"
  PreScanLaneMarker2/1 -> Subsystem/2(LaneMarkerInfo1)
  Subsystem/8(Lane4_Y) -> MATLAB Function/8(Lane4_Y)
  Demux3/1 -> Bus Creator/9  "Lane3C0"
  Demux1/4 -> Bus Creator/4  "Lane1C3"
  Demux3/2 -> Bus Creator/10  "Lane3C1"
  Demux4/2 -> Bus Creator/14  "Lane4C1"
  Demux1/1 -> Bus Creator/1  "Lane1C0"
  Demux2/1 -> Bus Creator/5  "Lane2C0"
  Subsystem/2(Lane3_Y) -> MATLAB Function/2(Lane3_Y)
  MATLAB Function/1(Lane1) -> Demux1/1
  MATLAB Function/2(Lane2) -> Demux2/1
  Subsystem/6(Lane2_Y) -> MATLAB Function/6(Lane2_Y)
  Subsystem/7(Lane4_X) -> MATLAB Function/7(Lane4_X)
  Subsystem/1(Lane3_X) -> MATLAB Function/1(Lane3_X)
  MATLAB Function/4(Lane4) -> Demux4/1
  MATLAB Function/3(Lane3) -> Demux3/1
  Subsystem/3(Lane1_X) -> MATLAB Function/3(Lane1_X)
  Subsystem/4(Lane1_Y) -> MATLAB Function/4(Lane1_Y)

== system DvrSimKeybdCircuit_cs/Roewe_550_S_Sedan_1/CarSim_Vehicle/CarSim2PreScanSTATE ==
  CarSim_In : Inport
  D2R : Gain  Gain=pi/180
  Demux : Demux  Outputs=[3 3 3 -1]
  Demux1 : Demux  Outputs=3
  Demux2 : Demux  Outputs=3
  Demux3 : Demux  Outputs=3
  Terminator : Terminator
  Transformation_SprungMassCarSim2PreScan : Subsystem
  km|h_to_m|s : Gain  Gain=1/3.6
  x [m] : Outport
  y [m] : Outport  Port=2
  z [m] : Outport  Port=3
  dx [m/s] : Outport  Port=4
  dy [m/s] : Outport  Port=5
  dz [m/s] : Outport  Port=6
  R [rad] : Outport  Port=7
  P [rad] : Outport  Port=8
  Y [rad] : Outport  Port=9
  wires:
  Demux/4 -> Terminator/1
  Demux3/3 -> Y [rad]/1
  Demux3/2 -> P [rad]/1
  Demux3/1 -> R [rad]/1
  Demux2/3 -> dz [m/s]/1
  Demux2/2 -> dy [m/s]/1
  Demux2/1 -> dx [m/s]/1
  Demux1/3 -> z [m]/1
  Demux1/2 -> y [m]/1
  Demux1/1 -> x [m]/1
  Transformation_SprungMassCarSim2PreScan/1(Out1) -> Demux1/1
  Demux/1 -> Transformation_SprungMassCarSim2PreScan/1(In1)
  CarSim_In/1 -> Demux/1
  km|h_to_m|s/1 -> Demux2/1
  Demux/2 -> km|h_to_m|s/1
  Demux/3 -> D2R/1
  D2R/1 -> Demux3/1

== system DvrSimKeybdCircuit_cs/Roewe_550_S_Sedan_1/CarSim_Vehicle/CarSim2PreScan_BUS ==
  CarSim_In : Inport
  Bus Creator2 : BusCreator  Inputs=3
  Bus Creator9 : BusCreator  Inputs=1
  Demux : Demux  Outputs=[3 3 3 12 12 2]
  Steering : Subsystem
  Vehicle : Subsystem
  Wheel : Subsystem
  PreScanBUS_VehicleDynamics : Outport
  wires:
  Steering/1(Steering) -> Bus Creator2/3
  Demux/6 -> Steering/1(SteeringWheel_In)  "SteeringWheel_In"
  CarSim_In/1 -> Demux/1
  Demux/1 -> Wheel/1(SprungMass_Pos_Global[x;y;z][m])  "SprungMass_Pos_Global[x;y;z][m]"
  Demux/5 -> Wheel/4(CarSim_Angle_Wheel_[FL;FR;RL;RR][x;y;z][deg;rev;deg])  "CarSim_Angle_Wheel_[FL;FR;RL;RR][x;y;z][deg;rev;deg]"
  Demux/4 -> Wheel/3(CarSim_Pos_Wheel_[FL;FR;RL;RR][x;y;z][m])  "CarSim_Pos_Wheel_[FL;FR;RL;RR][x;y;z][m]"
  Demux/3 -> Wheel/2(SprungMass_Angle_Global[x;y;z][deg])  "SprungMass_Angle_Global[x;y;z][deg]"
  Demux/2 -> Vehicle/1(v_VehicleCoG[x;y;z][km|h])  "v_VehicleCoG[x;y;z][km|h]"
  Wheel/1(Wheel) -> Bus Creator2/2
  Vehicle/1(Vehicle) -> Bus Creator2/1
  Bus Creator9/1 -> PreScanBUS_VehicleDynamics/1
  Bus Creator2/1 -> Bus Creator9/1  "PreScanBUS_VehicleDynamics"

== system DvrSimKeybdCircuit_cs/Roewe_550_S_Sedan_1/CarSim_Vehicle/CarSim2PreScan_ContactAdapter ==
  State : Inport
  State_Bus : Inport  Port=2
  Bus Selector : BusSelector  OutputSignals=PreScanBUS_VehicleDynamics.Vehicle.Velocities.Linear,PreScanBUS_VehicleDynamics.Wheel.Position.Linear
  Constant : Constant  Value=[ wheelRadius wheelRadius wheelRadius wheelRadius ]
  Embedded MATLAB Function : MATLAB Function  TreatAsAtomicUnit=on
  Memory : Memory
  Mux : Mux  Inputs="[9 1 12  4]"
  ContactParams : Outport
  wires:
  Memory/1 -> ContactParams/1
  Constant/1 -> Mux/4
  Bus Selector/1 -> Embedded MATLAB Function/1(u)  "<Linear>"
  State_Bus/1 -> Bus Selector/1
  Bus Selector/2 -> Mux/3  "<Linear>"
  State/1 -> Mux/1
  Embedded MATLAB Function/1(y) -> Mux/2
  Mux/1 -> Memory/1

== system DvrSimKeybdCircuit_cs/Roewe_550_S_Sedan_1/CarSim_Vehicle/MuxState ==
  note: mode: Dynamics
  note: mode: Positioning
  note: mode: Dynamics
      | VelVEHICLE
      | wrt VEH
  note: AnglesVEHICLE
      | wrtGLOB
  note: For state mode 'Dynamic' positions
      | are not taken into account, as they
      | are computed by integrating velocity.
      | Click annotation for Help.
  x [m] : Inport  SampleTime=TimeStep
  y [m] : Inport  Port=2  SampleTime=TimeStep
  z [m] : Inport  Port=3  SampleTime=TimeStep
  dx [m/s] : Inport  Port=4  SampleTime=TimeStep
  dy [m/s] : Inport  Port=5  SampleTime=TimeStep
  dz [m/s] : Inport  Port=6  SampleTime=TimeStep
  R [rad] : Inport  Port=7  SampleTime=TimeStep
  P [rad] : Inport  Port=8  SampleTime=TimeStep
  Y [rad] : Inport  Port=9  SampleTime=TimeStep
  Constant : Constant  DisableCoverage=on  Value=positioningmode
  Discrete-Time Integrator : DiscreteIntegrator  SampleTime=TimeStep  ICPrevOutput=DiscIntNeverNeededParam  ICPrevScaledInput=DiscIntNeverNeededParam
  Ground : Ground
  Ground1 : Ground
  Mux1 : Mux  Inputs=[3 3]
  Mux2 : Mux  Inputs=3
  Mux3 : Mux  Inputs=3
  Mux4 : Mux  Inputs=3
  Mux5 : Mux  Inputs=[3 3]
  Mux6 : Mux  Inputs=[6 3]
  Switch : Switch  Threshold=0.5
  Transformation_BODY2GLOBAL : PreScanSimulinkLibrary/Simple_Vehicle_Dynamics/Chassis/MuxDynState/Transformation_BODY2GLOBAL
  mux3 : Mux  Inputs=3
  state : Outport
  wires:
  Constant/1 -> Switch/2
  Mux6/1 -> state/1
  Mux4/1 -> Mux1/1
  Mux5/1 -> Switch/3
  Mux1/1 -> Switch/1
  Switch/1 -> Mux6/1  "PosVeh wrt  GLOB"
  P [rad]/1 -> Mux3/2
  R [rad]/1 -> Mux3/1
  dz [m/s]/1 -> Mux2/3
  dy [m/s]/1 -> Mux2/2
  dx [m/s]/1 -> Mux2/1
  z [m]/1 -> Mux4/3
  y [m]/1 -> Mux4/2
  x [m]/1 -> Mux4/1
  Ground1/1 -> mux3/2  "pitch"
  Y [rad]/1 -> mux3/3, Mux3/3  "yaw"
  Mux3/1 -> Mux6/2
  Transformation_BODY2GLOBAL/1 -> Discrete-Time Integrator/1, Mux5/2  "VelVEH wrt  GLOB"
  mux3/1 -> Transformation_BODY2GLOBAL/2
  Ground/1 -> mux3/1  "roll"
  Mux2/1 -> Mux1/2, Transformation_BODY2GLOBAL/1
  Discrete-Time Integrator/1 -> Mux5/1  "PosVEH wrt  GLOB"

== system DvrSimKeybdCircuit_cs/Roewe_550_S_Sedan_1/CarSim_Vehicle/TyreContact To Road Information ==
  TyreInfo_in : Inport
  Bus Selector3 : BusSelector  OutputSignals=TireFL.normal.x,TireFL.normal.y,TireFL.normal.z,TireFL.position.z,TireFR.normal.x,TireFR.normal.y,TireFR.normal.z,TireFR.position.z,TireRL.normal.x,TireRL.normal.y,TireRL.normal.z,TireRL.position.z,TireRR.normal.x,TireRR.normal.y,TireRR.normal.z,TireRR.position.z
  Contact To Road Information : Subsystem
  RoadSlopeAndZ_[FL;FR;RL;RR] : Outport
  wires:
  Bus Selector3/8 -> Contact To Road Information/8(" Pos_z_CP_CoorSys_E[FR]m]")  "<z>"
  Bus Selector3/7 -> Contact To Road Information/7(UnitVec_z_CP_CoorSys_E[FR][z])  "<z>"
  Contact To Road Information/1(RoadSlopeAndZ_[FL;FR;RL;RR]) -> RoadSlopeAndZ_[FL;FR;RL;RR]/1
  Bus Selector3/16 -> Contact To Road Information/16(" Pos_z_CP_CoorSys_E[RR]m]")  "<z>"
  Bus Selector3/15 -> Contact To Road Information/15(UnitVec_z_CP_CoorSys_E[RR][z])  "<z>"
  Bus Selector3/14 -> Contact To Road Information/14(UnitVec_z_CP_CoorSys_E[RR][y])  "<y>"
  Bus Selector3/13 -> Contact To Road Information/13(UnitVec_z_CP_CoorSys_E[RR][x])  "<x>"
  Bus Selector3/12 -> Contact To Road Information/12(" Pos_z_CP_CoorSys_E[RL]m]")  "<z>"
  Bus Selector3/11 -> Contact To Road Information/11(UnitVec_z_CP_CoorSys_E[RL][z])  "<z>"
  Bus Selector3/10 -> Contact To Road Information/10(UnitVec_z_CP_CoorSys_E[RL][y])  "<y>"
  Bus Selector3/9 -> Contact To Road Information/9(UnitVec_z_CP_CoorSys_E[RL][x])  "<x>"
  Bus Selector3/6 -> Contact To Road Information/6(UnitVec_z_CP_CoorSys_E[FR][y])  "<y>"
  Bus Selector3/5 -> Contact To Road Information/5(UnitVec_z_CP_CoorSys_E[FR][x])  "<x>"
  Bus Selector3/4 -> Contact To Road Information/4(" Pos_z_CP_CoorSys_E[FL]m]")  "<z>"
  Bus Selector3/3 -> Contact To Road Information/3(UnitVec_z_CP_CoorSys_E[FL][z])  "<z>"
  Bus Selector3/2 -> Contact To Road Information/2(UnitVec_z_CP_CoorSys_E[FL][y])  "<y>"
  Bus Selector3/1 -> Contact To Road Information/1(UnitVec_z_CP_CoorSys_E[FL][x])  "<x>"
  TyreInfo_in/1 -> Bus Selector3/1

== system DvrSimKeybdCircuit_cs/Roewe_550_S_Sedan_1/LaneMarkerSensor_1_Data/If Action Subsystem1 ==
  In1 : Inport
  In2 : Inport  Port=2
  Action Port : ActionPort  ActionType=then
  Bus Selector : BusSelector  OutputSignals=DATA
  Selector : Selector  IndexOptions=Index vector (port)  Indices=[4]  OutputSizes=1
  Out1 : Outport
  wires:
  Bus Selector/1 -> Out1/1  "<DATA>"
  Selector/1 -> Bus Selector/1
  In1/1 -> Selector/1
  In2/1 -> Selector/2

== system DvrSimKeybdCircuit_cs/Roewe_550_S_Sedan_1/LaneMarkerSensor_1_Data/If Action Subsystem2 ==
  In1 : Inport
  In2 : Inport  Port=2
  Action Port : ActionPort  ActionType=then
  Bus Selector : BusSelector  OutputSignals=DATA
  Selector : Selector  IndexOptions=Index vector (port)  Indices=[4]  OutputSizes=1
  Out1 : Outport
  wires:
  Bus Selector/1 -> Out1/1  "<DATA>"
  Selector/1 -> Bus Selector/1
  In1/1 -> Selector/1
  In2/1 -> Selector/2

== system DvrSimKeybdCircuit_cs/Roewe_550_S_Sedan_1/LaneMarkerSensor_1_Data/If Action Subsystem3 ==
  In1 : Inport
  In2 : Inport  Port=2
  Action Port : ActionPort  ActionType=then
  Bus Selector : BusSelector  OutputSignals=DATA
  Selector : Selector  IndexOptions=Index vector (port)  Indices=[4]  OutputSizes=1
  Out1 : Outport
  wires:
  Bus Selector/1 -> Out1/1  "<DATA>"
  Selector/1 -> Bus Selector/1
  In1/1 -> Selector/1
  In2/1 -> Selector/2

== system DvrSimKeybdCircuit_cs/Roewe_550_S_Sedan_1/LaneMarkerSensor_1_Data/If Action Subsystem4 ==
  In1 : Inport
  In2 : Inport  Port=2
  Action Port : ActionPort  ActionType=then
  Bus Selector : BusSelector  OutputSignals=DATA
  Selector : Selector  IndexOptions=Index vector (port)  Indices=[4]  OutputSizes=1
  Out1 : Outport
  wires:
  Bus Selector/1 -> Out1/1  "<DATA>"
  Selector/1 -> Bus Selector/1
  In1/1 -> Selector/1
  In2/1 -> Selector/2

== system DvrSimKeybdCircuit_cs/Roewe_550_S_Sedan_1/LaneMarkerSensor_2_Data/If Action Subsystem1 ==
  In1 : Inport
  In2 : Inport  Port=2
  Action Port : ActionPort  ActionType=then
  Bus Selector : BusSelector  OutputSignals=DATA
  Selector : Selector  IndexOptions=Index vector (port)  Indices=[4]  OutputSizes=1
  Out1 : Outport
  wires:
  Bus Selector/1 -> Out1/1  "<DATA>"
  Selector/1 -> Bus Selector/1
  In1/1 -> Selector/1
  In2/1 -> Selector/2

== system DvrSimKeybdCircuit_cs/Roewe_550_S_Sedan_1/LaneMarkerSensor_2_Data/If Action Subsystem2 ==
  In1 : Inport
  In2 : Inport  Port=2
  Action Port : ActionPort  ActionType=then
  Bus Selector : BusSelector  OutputSignals=DATA
  Selector : Selector  IndexOptions=Index vector (port)  Indices=[4]  OutputSizes=1
  Out1 : Outport
  wires:
  Bus Selector/1 -> Out1/1  "<DATA>"
  Selector/1 -> Bus Selector/1
  In1/1 -> Selector/1
  In2/1 -> Selector/2

== system DvrSimKeybdCircuit_cs/Roewe_550_S_Sedan_1/LaneMarkerSensor_2_Data/If Action Subsystem3 ==
  In1 : Inport
  In2 : Inport  Port=2
  Action Port : ActionPort  ActionType=then
  Bus Selector : BusSelector  OutputSignals=DATA
  Selector : Selector  IndexOptions=Index vector (port)  Indices=[4]  OutputSizes=1
  Out1 : Outport
  wires:
  Bus Selector/1 -> Out1/1  "<DATA>"
  Selector/1 -> Bus Selector/1
  In1/1 -> Selector/1
  In2/1 -> Selector/2

== system DvrSimKeybdCircuit_cs/Roewe_550_S_Sedan_1/LaneMarkerSensor_2_Data/If Action Subsystem4 ==
  In1 : Inport
  In2 : Inport  Port=2
  Action Port : ActionPort  ActionType=then
  Bus Selector : BusSelector  OutputSignals=DATA
  Selector : Selector  IndexOptions=Index vector (port)  Indices=[4]  OutputSizes=1
  Out1 : Outport
  wires:
  Bus Selector/1 -> Out1/1  "<DATA>"
  Selector/1 -> Bus Selector/1
  In1/1 -> Selector/1
  In2/1 -> Selector/2

== system DvrSimKeybdCircuit_cs/Roewe_550_S_Sedan_1/LaneMarkerSensor_3_Data/If Action Subsystem1 ==
  In1 : Inport
  In2 : Inport  Port=2
  Action Port : ActionPort  ActionType=then
  Bus Selector : BusSelector  OutputSignals=DATA
  Selector : Selector  IndexOptions=Index vector (port)  Indices=[4]  OutputSizes=1
  Out1 : Outport
  wires:
  Bus Selector/1 -> Out1/1  "<DATA>"
  Selector/1 -> Bus Selector/1
  In1/1 -> Selector/1
  In2/1 -> Selector/2

== system DvrSimKeybdCircuit_cs/Roewe_550_S_Sedan_1/LaneMarkerSensor_3_Data/If Action Subsystem2 ==
  In1 : Inport
  In2 : Inport  Port=2
  Action Port : ActionPort  ActionType=then
  Bus Selector : BusSelector  OutputSignals=DATA
  Selector : Selector  IndexOptions=Index vector (port)  Indices=[4]  OutputSizes=1
  Out1 : Outport
  wires:
  Bus Selector/1 -> Out1/1  "<DATA>"
  Selector/1 -> Bus Selector/1
  In1/1 -> Selector/1
  In2/1 -> Selector/2

== system DvrSimKeybdCircuit_cs/Roewe_550_S_Sedan_1/LaneMarkerSensor_3_Data/If Action Subsystem3 ==
  In1 : Inport
  In2 : Inport  Port=2
  Action Port : ActionPort  ActionType=then
  Bus Selector : BusSelector  OutputSignals=DATA
  Selector : Selector  IndexOptions=Index vector (port)  Indices=[4]  OutputSizes=1
  Out1 : Outport
  wires:
  Bus Selector/1 -> Out1/1  "<DATA>"
  Selector/1 -> Bus Selector/1
  In1/1 -> Selector/1
  In2/1 -> Selector/2

== system DvrSimKeybdCircuit_cs/Roewe_550_S_Sedan_1/LaneMarkerSensor_3_Data/If Action Subsystem4 ==
  In1 : Inport
  In2 : Inport  Port=2
  Action Port : ActionPort  ActionType=then
  Bus Selector : BusSelector  OutputSignals=DATA
  Selector : Selector  IndexOptions=Index vector (port)  Indices=[4]  OutputSizes=1
  Out1 : Outport
  wires:
  Bus Selector/1 -> Out1/1  "<DATA>"
  Selector/1 -> Bus Selector/1
  In1/1 -> Selector/1
  In2/1 -> Selector/2

== system DvrSimKeybdCircuit_cs/Roewe_550_S_Sedan_1/LaneMarkerSensor_4_Data/If Action Subsystem1 ==
  In1 : Inport
  In2 : Inport  Port=2
  Action Port : ActionPort  ActionType=then
  Bus Selector : BusSelector  OutputSignals=DATA
  Selector : Selector  IndexOptions=Index vector (port)  Indices=[4]  OutputSizes=1
  Out1 : Outport
  wires:
  Bus Selector/1 -> Out1/1  "<DATA>"
  Selector/1 -> Bus Selector/1
  In1/1 -> Selector/1
  In2/1 -> Selector/2
